simulink model "carga_HDLGEN"  (R2018a)
settings: Solver=FixedStepDiscrete  StartTime=0.0  StopTime=.2  FixedStep=1e-4  RelTol=1e-3
InitFcn:
  | Hs = tf([520 0], [1.3801 104 100]);
  | Hz = c2d(Hs, 1e-4, 'impulse');
settings Model: DataTypeOverride=Off  FPTRunName=Ranges(Double)  Creator=erich  LastModifiedBy=erich
settings DataIOCC: SaveOutput=off  SaveTime=off
settings OptimizationCC: BlockReduction=off  ConditionallyExecuteInputs=off  DefaultParameterBehavior=Inlined
settings DebuggingCC: AlgebraicLoopMsg=error  SingleTaskRateTransMsg=error  StrictBusMsg=ErrorOnBusTreatedAsVector
settings HardwareCC: ProdBitPerPointer=32  ProdBitPerSizeT=32  ProdBitPerPtrDiffT=32  ProdLargestAtomicFloat=None  ProdIntDivRoundTo=Undefined  ProdEndianess=Unspecified  ProdWordSize=32  ProdHWDeviceType=ASIC/FPGA->ASIC/FPGA  ProdEqTarget=off
settings CodeAppCC: StateflowObjectComments=on
settings GRTTargetCC: TargetLangStandard=C89/C90 (ANSI)

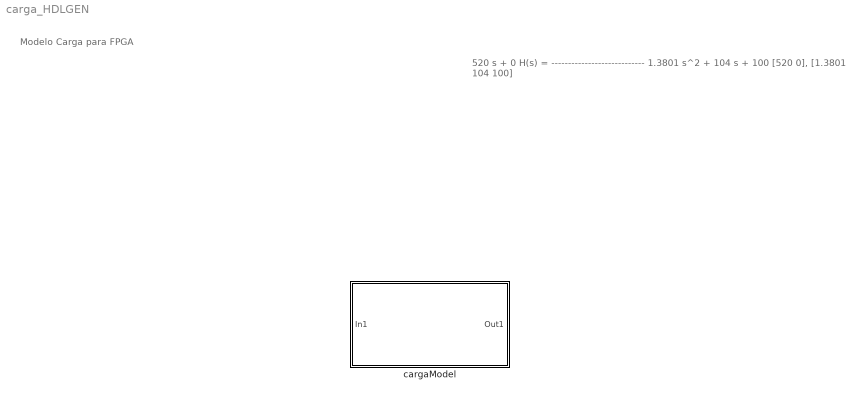
== system carga_HDLGEN ==
  note: 520 s + 0
      | H(s) = ----------------------------
      | 1.3801 s^2 + 104 s + 100
      |
      | [520 0], [1.3801 104 100]
  note: Modelo Carga
      | para FPGA
  cargaModel : Subsystem

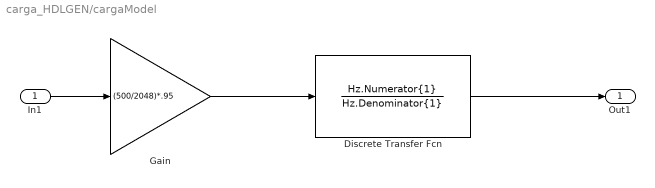
== system carga_HDLGEN/cargaModel ==
  In1 : Inport  OutDataTypeStr=int16
  Discrete Transfer Fcn : DiscreteTransferFcn  Numerator=Hz.Numerator{1}  Denominator=Hz.Denominator{1}  SampleTime=1e-4  StateDataTypeStr=int32  NumCoefDataTypeStr=fixdt(1,32,28)  DenCoefDataTypeStr=fixdt(1,32,28)  NumProductDataTypeStr=fixdt(1,32,10)  DenProductDataTypeStr=fixdt(1,32,10)  NumAccumDataTypeStr=fixdt(1,32,10)  DenAccumDataTypeStr=fixdt(1,32,10)  OutDataTypeStr=int16  RndMeth=Round
  Gain : Gain  Gain=(500/2048)*.95  ParamDataTypeStr=fixdt(1,32,10)
  Out1 : Outport  OutDataTypeStr=int16
  wires:
  Discrete Transfer Fcn/1 -> Out1/1
  In1/1 -> Gain/1
  Gain/1 -> Discrete Transfer Fcn/1
